simulink subsystem "RoboticArmGeneral7DOF_2"  (R2023a)
settings: Solver=VariableStepAuto  StartTime=0.0  StopTime=10.0  RelTol=1e-3
model mask{armAttach_Data=0, joint1_Data=0, joint2_Data=0, joint3_Data=0, joint4_Data=0, joint5_Data=0, joint6_Data=0, joint7_Data=0, ee_State_Data=0}
undefined symbols (not defined in the file or in its folder): arm, X, Y, Z
libraries: sm_lib x62, nesl_utility x35
(part 2 of 2)

== system RoboticArmGeneral7DOF_2/ElbowAssem_1/MainLink2_1_RIGID ==
  ReferenceFrame : sm_lib/Frames and Transforms/Reference Frame
  Solid : sm_lib/Body Elements/File Solid  ExtGeomFileName=MainLink2_Default_sldprt.STEP  UnitType=FromFile  ExtGeomFileUnits=m  StepReaderType=HEX  ExportConvexHullGeometry=off  InertiaType=Custom  Mass=arm(2).smiData.Solid(3).mass  MassUnits=kg  CenterOfMass=arm(2).smiData.Solid(3).CoM  CenterOfMassUnits=m  MomentsOfInertia=arm(2).smiData.Solid(3).MoI  MomentsOfInertiaUnits=kg*m^2  ProductsOfInertia=arm(2).smiData.Solid(3).PoI  ProductsOfInertiaUnits=kg*m^2  BasedOnType=DensityFromFile  Density=1000  DensityUnits=kg/m^3  DoExposeReferenceFrame=on  SerializedFrames=<Frames/>  GraphicType=FromGeometry  MarkerShape=Sphere  MarkerSize=10  GraphicVisPropType=SimpleVisualProperties  GraphicDiffuseColor=arm(2).smiData.Solid(3).color  GraphicSpecularColor=[0.5 0.5 0.5 1.0]  GraphicAmbientColor=[0.15 0.15 0.15 1.0]  GraphicEmissiveColor=[0.0 0.0 0.0 1.0]  GraphicShininess=75  GraphicOpacity=arm(2).smiData.Solid(3).opacity
  Transform : sm_lib/Frames and Transforms/Rigid Transform  TranslationMethod=Cartesian  TranslationStandardOffset=0  TranslationStandardOffsetUnits=m  TranslationStandardAxis=+Z  TranslationCartesianOffset=arm(2).smiData.RigidTransform(5).translation  TranslationCartesianOffsetUnits=m  TranslationROffset=0  TranslationROffsetUnits=m  TranslationZOffset=0  TranslationZOffsetUnits=m  TranslationThetaOffset=0  TranslationThetaOffsetUnits=deg  RotationMethod=ArbitraryAxis  RotationAngleUnits=rad  RotationStandardAxis=+Z  RotationAngle=arm(2).smiData.RigidTransform(5).angle  RotationArbitraryAxis=arm(2).smiData.RigidTransform(5).axis  FollAlignAxisA=+X  BaseAlignAxisA=+Y  FollAlignAxisB=+Y  BaseAlignAxisB=+Z  RotationSequenceAxes=FollowerAxes  RotationSequence=XYX  RotationSequenceAngles=[0 0 0]  RotationSequenceAnglesUnits=deg  RotationMatrix=[1 0 0; 0 1 0; 0 0 1]  Quaternion=[1 0 0 0]
  Transform1 : sm_lib/Frames and Transforms/Rigid Transform  TranslationMethod=Cartesian  TranslationStandardOffset=0  TranslationStandardOffsetUnits=m  TranslationStandardAxis=+Z  TranslationCartesianOffset=arm(2).smiData.RigidTransform(19).translation  TranslationCartesianOffsetUnits=m  TranslationROffset=0  TranslationROffsetUnits=m  TranslationZOffset=0  TranslationZOffsetUnits=m  TranslationThetaOffset=0  TranslationThetaOffsetUnits=deg  RotationMethod=ArbitraryAxis  RotationAngleUnits=rad  RotationStandardAxis=+Z  RotationAngle=arm(2).smiData.RigidTransform(19).angle  RotationArbitraryAxis=arm(2).smiData.RigidTransform(19).axis  FollAlignAxisA=+X  BaseAlignAxisA=+Y  FollAlignAxisB=+Y  BaseAlignAxisB=+Z  RotationSequenceAxes=FollowerAxes  RotationSequence=XYX  RotationSequenceAngles=[0 0 0]  RotationSequenceAnglesUnits=deg  RotationMatrix=[1 0 0; 0 1 0; 0 0 1]  Quaternion=[1 0 0 0]
  MainLink_End : PMIOPort  Side=Right
  J5_2 : PMIOPort  Port=2  Side=Left
  connections:
  Transform1/RConn1 -- MainLink_End/RConn1
  Transform/RConn1 -- J5_2/RConn1
  Transform1/LConn1 -- Transform/LConn1 -- ReferenceFrame/RConn1 -- Solid/RConn1

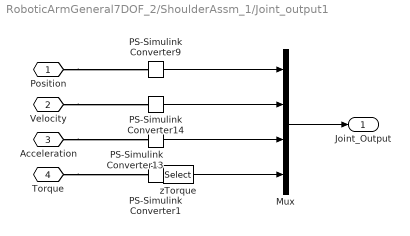
== system RoboticArmGeneral7DOF_2/ShoulderAssm_1/Joint_output1 ==
  Mux : Mux
  PS-Simulink Converter{1,9,13..14} (4 alike) : nesl_utility/PS-Simulink Converter  PhysicalDomain=network_engine_domain  SubClassName=ps_output  LeftPortType=input  RightPortType=output  PseudoPeriodic=off  Frequencies=[]  VectorFormat=1-D array  Unit=inherit  AffineConversion=off
  zTorque : Selector  InputPortWidth=3  IndexOptions=Index vector (dialog)  Indices=3  OutputSizes=1
  Position : PMIOPort  Side=Left
  Velocity : PMIOPort  Port=2  Side=Left
  Acceleration : PMIOPort  Port=3  Side=Left
  Torque : PMIOPort  Port=4  Side=Left
  Joint_Output : Outport
  wires:
  PS-Simulink Converter1/1 -> zTorque/1
  PS-Simulink Converter13/1 -> Mux/3
  PS-Simulink Converter9/1 -> Mux/1
  zTorque/1 -> Mux/4
  PS-Simulink Converter14/1 -> Mux/2
  Mux/1 -> Joint_Output/1
  connections:
  Position/RConn1 -- PS-Simulink Converter9/LConn1
  Acceleration/RConn1 -- PS-Simulink Converter13/LConn1
  Torque/RConn1 -- PS-Simulink Converter1/LConn1
  Velocity/RConn1 -- PS-Simulink Converter14/LConn1

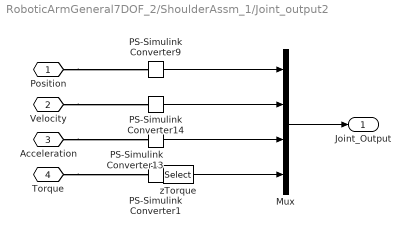
== system RoboticArmGeneral7DOF_2/ShoulderAssm_1/Joint_output2 ==
  Mux : Mux
  PS-Simulink Converter{1,9,13..14} (4 alike) : nesl_utility/PS-Simulink Converter  PhysicalDomain=network_engine_domain  SubClassName=ps_output  LeftPortType=input  RightPortType=output  PseudoPeriodic=off  Frequencies=[]  VectorFormat=1-D array  Unit=inherit  AffineConversion=off
  zTorque : Selector  InputPortWidth=3  IndexOptions=Index vector (dialog)  Indices=3  OutputSizes=1
  Position : PMIOPort  Side=Left
  Velocity : PMIOPort  Port=2  Side=Left
  Acceleration : PMIOPort  Port=3  Side=Left
  Torque : PMIOPort  Port=4  Side=Left
  Joint_Output : Outport
  wires:
  PS-Simulink Converter1/1 -> zTorque/1
  PS-Simulink Converter13/1 -> Mux/3
  PS-Simulink Converter9/1 -> Mux/1
  zTorque/1 -> Mux/4
  PS-Simulink Converter14/1 -> Mux/2
  Mux/1 -> Joint_Output/1
  connections:
  Position/RConn1 -- PS-Simulink Converter9/LConn1
  Acceleration/RConn1 -- PS-Simulink Converter13/LConn1
  Torque/RConn1 -- PS-Simulink Converter1/LConn1
  Velocity/RConn1 -- PS-Simulink Converter14/LConn1

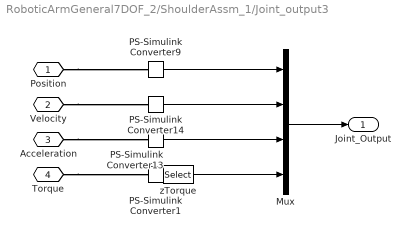
== system RoboticArmGeneral7DOF_2/ShoulderAssm_1/Joint_output3 ==
  Mux : Mux
  PS-Simulink Converter{1,9,13..14} (4 alike) : nesl_utility/PS-Simulink Converter  PhysicalDomain=network_engine_domain  SubClassName=ps_output  LeftPortType=input  RightPortType=output  PseudoPeriodic=off  Frequencies=[]  VectorFormat=1-D array  Unit=inherit  AffineConversion=off
  zTorque : Selector  InputPortWidth=3  IndexOptions=Index vector (dialog)  Indices=3  OutputSizes=1
  Position : PMIOPort  Side=Left
  Velocity : PMIOPort  Port=2  Side=Left
  Acceleration : PMIOPort  Port=3  Side=Left
  Torque : PMIOPort  Port=4  Side=Left
  Joint_Output : Outport
  wires:
  PS-Simulink Converter1/1 -> zTorque/1
  PS-Simulink Converter13/1 -> Mux/3
  PS-Simulink Converter9/1 -> Mux/1
  zTorque/1 -> Mux/4
  PS-Simulink Converter14/1 -> Mux/2
  Mux/1 -> Joint_Output/1
  connections:
  Position/RConn1 -- PS-Simulink Converter9/LConn1
  Acceleration/RConn1 -- PS-Simulink Converter13/LConn1
  Torque/RConn1 -- PS-Simulink Converter1/LConn1
  Velocity/RConn1 -- PS-Simulink Converter14/LConn1

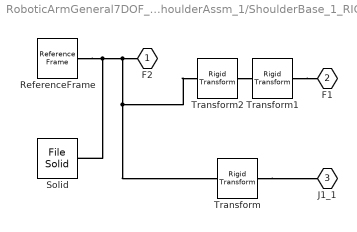
== system RoboticArmGeneral7DOF_2/ShoulderAssm_1/ShoulderBase_1_RIGID ==
  ReferenceFrame : sm_lib/Frames and Transforms/Reference Frame
  Solid : sm_lib/Body Elements/File Solid  ExtGeomFileName=ShoulderBase_Default_sldprt.STEP  UnitType=FromFile  ExtGeomFileUnits=m  StepReaderType=HEX  ExportConvexHullGeometry=off  InertiaType=Custom  Mass=arm(2).smiData.Solid(9).mass  MassUnits=kg  CenterOfMass=arm(2).smiData.Solid(9).CoM  CenterOfMassUnits=m  MomentsOfInertia=arm(2).smiData.Solid(9).MoI  MomentsOfInertiaUnits=kg*m^2  ProductsOfInertia=arm(2).smiData.Solid(9).PoI  ProductsOfInertiaUnits=kg*m^2  BasedOnType=DensityFromFile  Density=1000  DensityUnits=kg/m^3  DoExposeReferenceFrame=on  SerializedFrames=<Frames/>  GraphicType=FromGeometry  MarkerShape=Sphere  MarkerSize=10  GraphicVisPropType=SimpleVisualProperties  GraphicDiffuseColor=arm(2).smiData.Solid(9).color  GraphicSpecularColor=[0.5 0.5 0.5 1.0]  GraphicAmbientColor=[0.15 0.15 0.15 1.0]  GraphicEmissiveColor=[0.0 0.0 0.0 1.0]  GraphicShininess=75  GraphicOpacity=arm(2).smiData.Solid(9).opacity
  Transform : sm_lib/Frames and Transforms/Rigid Transform  TranslationMethod=Cartesian  TranslationStandardOffset=0  TranslationStandardOffsetUnits=m  TranslationStandardAxis=+Z  TranslationCartesianOffset=arm(2).smiData.RigidTransform(9).translation  TranslationCartesianOffsetUnits=m  TranslationROffset=0  TranslationROffsetUnits=m  TranslationZOffset=0  TranslationZOffsetUnits=m  TranslationThetaOffset=0  TranslationThetaOffsetUnits=deg  RotationMethod=ArbitraryAxis  RotationAngleUnits=rad  RotationStandardAxis=+Z  RotationAngle=arm(2).smiData.RigidTransform(9).angle  RotationArbitraryAxis=arm(2).smiData.RigidTransform(9).axis  FollAlignAxisA=+X  BaseAlignAxisA=+Y  FollAlignAxisB=+Y  BaseAlignAxisB=+Z  RotationSequenceAxes=FollowerAxes  RotationSequence=XYX  RotationSequenceAngles=[0 0 0]  RotationSequenceAnglesUnits=deg  RotationMatrix=[1 0 0; 0 1 0; 0 0 1]  Quaternion=[1 0 0 0]
  Transform1 : sm_lib/Frames and Transforms/Rigid Transform  TranslationMethod=Cartesian  TranslationStandardOffset=0  TranslationStandardOffsetUnits=m  TranslationStandardAxis=+Z  TranslationCartesianOffset=arm(2).smiData.RigidTransform(15).translation  TranslationCartesianOffsetUnits=m  TranslationROffset=0  TranslationROffsetUnits=m  TranslationZOffset=0  TranslationZOffsetUnits=m  TranslationThetaOffset=0  TranslationThetaOffsetUnits=deg  RotationMethod=ArbitraryAxis  RotationAngleUnits=rad  RotationStandardAxis=+Z  RotationAngle=arm(2).smiData.RigidTransform(15).angle  RotationArbitraryAxis=arm(2).smiData.RigidTransform(15).axis  FollAlignAxisA=+X  BaseAlignAxisA=+Y  FollAlignAxisB=+Y  BaseAlignAxisB=+Z  RotationSequenceAxes=FollowerAxes  RotationSequence=XYX  RotationSequenceAngles=[0 0 0]  RotationSequenceAnglesUnits=deg  RotationMatrix=[1 0 0; 0 1 0; 0 0 1]  Quaternion=[1 0 0 0]
  Transform2 : sm_lib/Frames and Transforms/Rigid Transform  TranslationMethod=Cartesian  TranslationStandardOffset=0  TranslationStandardOffsetUnits=m  TranslationStandardAxis=+Z  TranslationCartesianOffset=arm(2).smiData.RigidTransform(25).translation  TranslationCartesianOffsetUnits=m  TranslationROffset=0  TranslationROffsetUnits=m  TranslationZOffset=0  TranslationZOffsetUnits=m  TranslationThetaOffset=0  TranslationThetaOffsetUnits=deg  RotationMethod=ArbitraryAxis  RotationAngleUnits=rad  RotationStandardAxis=+Z  RotationAngle=arm(2).smiData.RigidTransform(25).angle  RotationArbitraryAxis=arm(2).smiData.RigidTransform(25).axis  FollAlignAxisA=+X  BaseAlignAxisA=+Y  FollAlignAxisB=+Y  BaseAlignAxisB=+Z  RotationSequenceAxes=FollowerAxes  RotationSequence=XYX  RotationSequenceAngles=[0 0 0]  RotationSequenceAnglesUnits=deg  RotationMatrix=[1 0 0; 0 1 0; 0 0 1]  Quaternion=[1 0 0 0]
  F2 : PMIOPort  Side=Left
  F1 : PMIOPort  Port=2  Side=Left
  J1_1 : PMIOPort  Port=3  Side=Right
  connections:
  Transform2/LConn1 -- Transform/LConn1 -- F2/RConn1 -- ReferenceFrame/RConn1 -- Solid/RConn1
  Transform1/RConn1 -- F1/RConn1
  Transform/RConn1 -- J1_1/RConn1
  Transform2/RConn1 -- Transform1/LConn1

== system RoboticArmGeneral7DOF_2/ShoulderAssm_1/ShoulderJoint_1_1_RIGID ==
  ReferenceFrame : sm_lib/Frames and Transforms/Reference Frame
  Solid : sm_lib/Body Elements/File Solid  ExtGeomFileName=ShoulderJoint_1_Default_sldprt.STEP  UnitType=FromFile  ExtGeomFileUnits=m  StepReaderType=HEX  ExportConvexHullGeometry=off  InertiaType=Custom  Mass=arm(2).smiData.Solid(7).mass  MassUnits=kg  CenterOfMass=arm(2).smiData.Solid(7).CoM  CenterOfMassUnits=m  MomentsOfInertia=arm(2).smiData.Solid(7).MoI  MomentsOfInertiaUnits=kg*m^2  ProductsOfInertia=arm(2).smiData.Solid(7).PoI  ProductsOfInertiaUnits=kg*m^2  BasedOnType=DensityFromFile  Density=1000  DensityUnits=kg/m^3  DoExposeReferenceFrame=on  SerializedFrames=<Frames/>  GraphicType=FromGeometry  MarkerShape=Sphere  MarkerSize=10  GraphicVisPropType=SimpleVisualProperties  GraphicDiffuseColor=arm(2).smiData.Solid(7).color  GraphicSpecularColor=[0.5 0.5 0.5 1.0]  GraphicAmbientColor=[0.15 0.15 0.15 1.0]  GraphicEmissiveColor=[0.0 0.0 0.0 1.0]  GraphicShininess=75  GraphicOpacity=arm(2).smiData.Solid(7).opacity
  Transform : sm_lib/Frames and Transforms/Rigid Transform  TranslationMethod=Cartesian  TranslationStandardOffset=0  TranslationStandardOffsetUnits=m  TranslationStandardAxis=+Z  TranslationCartesianOffset=arm(2).smiData.RigidTransform(10).translation  TranslationCartesianOffsetUnits=m  TranslationROffset=0  TranslationROffsetUnits=m  TranslationZOffset=0  TranslationZOffsetUnits=m  TranslationThetaOffset=0  TranslationThetaOffsetUnits=deg  RotationMethod=ArbitraryAxis  RotationAngleUnits=rad  RotationStandardAxis=+Z  RotationAngle=arm(2).smiData.RigidTransform(10).angle  RotationArbitraryAxis=arm(2).smiData.RigidTransform(10).axis  FollAlignAxisA=+X  BaseAlignAxisA=+Y  FollAlignAxisB=+Y  BaseAlignAxisB=+Z  RotationSequenceAxes=FollowerAxes  RotationSequence=XYX  RotationSequenceAngles=[0 0 0]  RotationSequenceAnglesUnits=deg  RotationMatrix=[1 0 0; 0 1 0; 0 0 1]  Quaternion=[1 0 0 0]
  Transform1 : sm_lib/Frames and Transforms/Rigid Transform  TranslationMethod=Cartesian  TranslationStandardOffset=0  TranslationStandardOffsetUnits=m  TranslationStandardAxis=+Z  TranslationCartesianOffset=arm(2).smiData.RigidTransform(11).translation  TranslationCartesianOffsetUnits=m  TranslationROffset=0  TranslationROffsetUnits=m  TranslationZOffset=0  TranslationZOffsetUnits=m  TranslationThetaOffset=0  TranslationThetaOffsetUnits=deg  RotationMethod=ArbitraryAxis  RotationAngleUnits=rad  RotationStandardAxis=+Z  RotationAngle=arm(2).smiData.RigidTransform(11).angle  RotationArbitraryAxis=arm(2).smiData.RigidTransform(11).axis  FollAlignAxisA=+X  BaseAlignAxisA=+Y  FollAlignAxisB=+Y  BaseAlignAxisB=+Z  RotationSequenceAxes=FollowerAxes  RotationSequence=XYX  RotationSequenceAngles=[0 0 0]  RotationSequenceAnglesUnits=deg  RotationMatrix=[1 0 0; 0 1 0; 0 0 1]  Quaternion=[1 0 0 0]
  Shoulder1 : PMIOPort  Side=Right
  J1_2 : PMIOPort  Port=2  Side=Left
  AfterT : PMIOPort  Port=3  Side=Left
  connections:
  Shoulder1/RConn1 -- Transform1/RConn1
  Transform/RConn1 -- J1_2/RConn1
  AfterT/RConn1 -- Transform1/LConn1 -- ReferenceFrame/RConn1 -- Solid/RConn1 -- Transform/LConn1

== system RoboticArmGeneral7DOF_2/ShoulderAssm_1/ShoulderJoint_2_1_RIGID ==
  ReferenceFrame : sm_lib/Frames and Transforms/Reference Frame
  Solid : sm_lib/Body Elements/File Solid  ExtGeomFileName=ShoulderJoint_2_Default_sldprt.STEP  UnitType=FromFile  ExtGeomFileUnits=m  StepReaderType=HEX  ExportConvexHullGeometry=off  InertiaType=Custom  Mass=arm(2).smiData.Solid(8).mass  MassUnits=kg  CenterOfMass=arm(2).smiData.Solid(8).CoM  CenterOfMassUnits=m  MomentsOfInertia=arm(2).smiData.Solid(8).MoI  MomentsOfInertiaUnits=kg*m^2  ProductsOfInertia=arm(2).smiData.Solid(8).PoI  ProductsOfInertiaUnits=kg*m^2  BasedOnType=DensityFromFile  Density=1000  DensityUnits=kg/m^3  DoExposeReferenceFrame=on  SerializedFrames=<Frames/>  GraphicType=FromGeometry  MarkerShape=Sphere  MarkerSize=10  GraphicVisPropType=SimpleVisualProperties  GraphicDiffuseColor=arm(2).smiData.Solid(8).color  GraphicSpecularColor=[0.5 0.5 0.5 1.0]  GraphicAmbientColor=[0.15 0.15 0.15 1.0]  GraphicEmissiveColor=[0.0 0.0 0.0 1.0]  GraphicShininess=75  GraphicOpacity=arm(2).smiData.Solid(8).opacity
  Transform : sm_lib/Frames and Transforms/Rigid Transform  TranslationMethod=Cartesian  TranslationStandardOffset=0  TranslationStandardOffsetUnits=m  TranslationStandardAxis=+Z  TranslationCartesianOffset=arm(2).smiData.RigidTransform(12).translation  TranslationCartesianOffsetUnits=m  TranslationROffset=0  TranslationROffsetUnits=m  TranslationZOffset=0  TranslationZOffsetUnits=m  TranslationThetaOffset=0  TranslationThetaOffsetUnits=deg  RotationMethod=ArbitraryAxis  RotationAngleUnits=rad  RotationStandardAxis=+Z  RotationAngle=arm(2).smiData.RigidTransform(12).angle  RotationArbitraryAxis=arm(2).smiData.RigidTransform(12).axis  FollAlignAxisA=+X  BaseAlignAxisA=+Y  FollAlignAxisB=+Y  BaseAlignAxisB=+Z  RotationSequenceAxes=FollowerAxes  RotationSequence=XYX  RotationSequenceAngles=[0 0 0]  RotationSequenceAnglesUnits=deg  RotationMatrix=[1 0 0; 0 1 0; 0 0 1]  Quaternion=[1 0 0 0]
  Transform1 : sm_lib/Frames and Transforms/Rigid Transform  TranslationMethod=Cartesian  TranslationStandardOffset=0  TranslationStandardOffsetUnits=m  TranslationStandardAxis=+Z  TranslationCartesianOffset=arm(2).smiData.RigidTransform(13).translation  TranslationCartesianOffsetUnits=m  TranslationROffset=0  TranslationROffsetUnits=m  TranslationZOffset=0  TranslationZOffsetUnits=m  TranslationThetaOffset=0  TranslationThetaOffsetUnits=deg  RotationMethod=ArbitraryAxis  RotationAngleUnits=rad  RotationStandardAxis=+Z  RotationAngle=arm(2).smiData.RigidTransform(13).angle  RotationArbitraryAxis=arm(2).smiData.RigidTransform(13).axis  FollAlignAxisA=+X  BaseAlignAxisA=+Y  FollAlignAxisB=+Y  BaseAlignAxisB=+Z  RotationSequenceAxes=FollowerAxes  RotationSequence=XYX  RotationSequenceAngles=[0 0 0]  RotationSequenceAnglesUnits=deg  RotationMatrix=[1 0 0; 0 1 0; 0 0 1]  Quaternion=[1 0 0 0]
  J2_1 : PMIOPort  Side=Right
  Shoulder1 : PMIOPort  Port=2  Side=Left
  connections:
  Transform1/RConn1 -- J2_1/RConn1
  Transform/RConn1 -- Shoulder1/RConn1
  Solid/RConn1 -- Transform1/LConn1 -- Transform/LConn1 -- ReferenceFrame/RConn1

== system RoboticArmGeneral7DOF_2/ShoulderAssm_1/ShoulderJoint_3_4_RIGID ==
  ReferenceFrame : sm_lib/Frames and Transforms/Reference Frame
  Solid : sm_lib/Body Elements/File Solid  ExtGeomFileName=ShoulderJoint_3_Default_sldprt.STEP  UnitType=FromFile  ExtGeomFileUnits=m  StepReaderType=HEX  ExportConvexHullGeometry=off  InertiaType=Custom  Mass=arm(2).smiData.Solid(10).mass  MassUnits=kg  CenterOfMass=arm(2).smiData.Solid(10).CoM  CenterOfMassUnits=m  MomentsOfInertia=arm(2).smiData.Solid(10).MoI  MomentsOfInertiaUnits=kg*m^2  ProductsOfInertia=arm(2).smiData.Solid(10).PoI  ProductsOfInertiaUnits=kg*m^2  BasedOnType=DensityFromFile  Density=1000  DensityUnits=kg/m^3  DoExposeReferenceFrame=on  SerializedFrames=<Frames/>  GraphicType=FromGeometry  MarkerShape=Sphere  MarkerSize=10  GraphicVisPropType=SimpleVisualProperties  GraphicDiffuseColor=arm(2).smiData.Solid(10).color  GraphicSpecularColor=[0.5 0.5 0.5 1.0]  GraphicAmbientColor=[0.15 0.15 0.15 1.0]  GraphicEmissiveColor=[0.0 0.0 0.0 1.0]  GraphicShininess=75  GraphicOpacity=arm(2).smiData.Solid(10).opacity
  Transform : sm_lib/Frames and Transforms/Rigid Transform  TranslationMethod=Cartesian  TranslationStandardOffset=0  TranslationStandardOffsetUnits=m  TranslationStandardAxis=+Z  TranslationCartesianOffset=arm(2).smiData.RigidTransform(14).translation  TranslationCartesianOffsetUnits=m  TranslationROffset=0  TranslationROffsetUnits=m  TranslationZOffset=0  TranslationZOffsetUnits=m  TranslationThetaOffset=0  TranslationThetaOffsetUnits=deg  RotationMethod=ArbitraryAxis  RotationAngleUnits=rad  RotationStandardAxis=+Z  RotationAngle=arm(2).smiData.RigidTransform(14).angle  RotationArbitraryAxis=arm(2).smiData.RigidTransform(14).axis  FollAlignAxisA=+X  BaseAlignAxisA=+Y  FollAlignAxisB=+Y  BaseAlignAxisB=+Z  RotationSequenceAxes=FollowerAxes  RotationSequence=XYX  RotationSequenceAngles=[0 0 0]  RotationSequenceAnglesUnits=deg  RotationMatrix=[1 0 0; 0 1 0; 0 0 1]  Quaternion=[1 0 0 0]
  Transform1 : sm_lib/Frames and Transforms/Rigid Transform  TranslationMethod=Cartesian  TranslationStandardOffset=0  TranslationStandardOffsetUnits=m  TranslationStandardAxis=+Z  TranslationCartesianOffset=arm(2).smiData.RigidTransform(21).translation  TranslationCartesianOffsetUnits=m  TranslationROffset=0  TranslationROffsetUnits=m  TranslationZOffset=0  TranslationZOffsetUnits=m  TranslationThetaOffset=0  TranslationThetaOffsetUnits=deg  RotationMethod=ArbitraryAxis  RotationAngleUnits=rad  RotationStandardAxis=+Z  RotationAngle=arm(2).smiData.RigidTransform(21).angle  RotationArbitraryAxis=arm(2).smiData.RigidTransform(21).axis  FollAlignAxisA=+X  BaseAlignAxisA=+Y  FollAlignAxisB=+Y  BaseAlignAxisB=+Z  RotationSequenceAxes=FollowerAxes  RotationSequence=XYX  RotationSequenceAngles=[0 0 0]  RotationSequenceAnglesUnits=deg  RotationMatrix=[1 0 0; 0 1 0; 0 0 1]  Quaternion=[1 0 0 0]
  J3_1 : PMIOPort  Side=Right
  J2_2 : PMIOPort  Port=2  Side=Left
  connections:
  Transform1/RConn1 -- J3_1/RConn1
  Transform/RConn1 -- J2_2/RConn1
  Transform1/LConn1 -- Transform/LConn1 -- ReferenceFrame/RConn1 -- Solid/RConn1

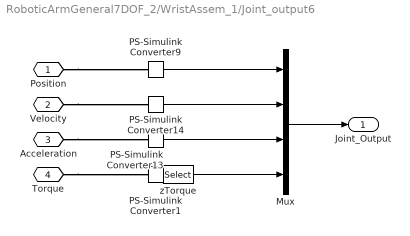
== system RoboticArmGeneral7DOF_2/WristAssem_1/Joint_output6 ==
  Mux : Mux
  PS-Simulink Converter{1,9,13..14} (4 alike) : nesl_utility/PS-Simulink Converter  PhysicalDomain=network_engine_domain  SubClassName=ps_output  LeftPortType=input  RightPortType=output  PseudoPeriodic=off  Frequencies=[]  VectorFormat=1-D array  Unit=inherit  AffineConversion=off
  zTorque : Selector  InputPortWidth=3  IndexOptions=Index vector (dialog)  Indices=3  OutputSizes=1
  Position : PMIOPort  Side=Left
  Velocity : PMIOPort  Port=2  Side=Left
  Acceleration : PMIOPort  Port=3  Side=Left
  Torque : PMIOPort  Port=4  Side=Left
  Joint_Output : Outport
  wires:
  PS-Simulink Converter1/1 -> zTorque/1
  PS-Simulink Converter13/1 -> Mux/3
  PS-Simulink Converter9/1 -> Mux/1
  zTorque/1 -> Mux/4
  PS-Simulink Converter14/1 -> Mux/2
  Mux/1 -> Joint_Output/1
  connections:
  Position/RConn1 -- PS-Simulink Converter9/LConn1
  Acceleration/RConn1 -- PS-Simulink Converter13/LConn1
  Torque/RConn1 -- PS-Simulink Converter1/LConn1
  Velocity/RConn1 -- PS-Simulink Converter14/LConn1

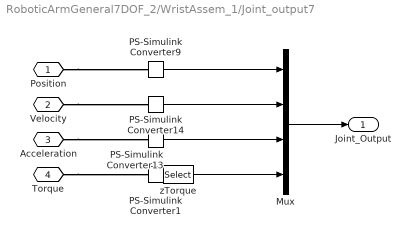
== system RoboticArmGeneral7DOF_2/WristAssem_1/Joint_output7 ==
  Mux : Mux
  PS-Simulink Converter{1,9,13..14} (4 alike) : nesl_utility/PS-Simulink Converter  PhysicalDomain=network_engine_domain  SubClassName=ps_output  LeftPortType=input  RightPortType=output  PseudoPeriodic=off  Frequencies=[]  VectorFormat=1-D array  Unit=inherit  AffineConversion=off
  zTorque : Selector  InputPortWidth=3  IndexOptions=Index vector (dialog)  Indices=3  OutputSizes=1
  Position : PMIOPort  Side=Left
  Velocity : PMIOPort  Port=2  Side=Left
  Acceleration : PMIOPort  Port=3  Side=Left
  Torque : PMIOPort  Port=4  Side=Left
  Joint_Output : Outport
  wires:
  PS-Simulink Converter1/1 -> zTorque/1
  PS-Simulink Converter13/1 -> Mux/3
  PS-Simulink Converter9/1 -> Mux/1
  zTorque/1 -> Mux/4
  PS-Simulink Converter14/1 -> Mux/2
  Mux/1 -> Joint_Output/1
  connections:
  Position/RConn1 -- PS-Simulink Converter9/LConn1
  Acceleration/RConn1 -- PS-Simulink Converter13/LConn1
  Torque/RConn1 -- PS-Simulink Converter1/LConn1
  Velocity/RConn1 -- PS-Simulink Converter14/LConn1

== system RoboticArmGeneral7DOF_2/WristAssem_1/WristJoint_1_1_RIGID ==
  ReferenceFrame : sm_lib/Frames and Transforms/Reference Frame
  Solid : sm_lib/Body Elements/File Solid  ExtGeomFileName=WristJoint_1_Default_sldprt.STEP  UnitType=FromFile  ExtGeomFileUnits=m  StepReaderType=HEX  ExportConvexHullGeometry=off  InertiaType=Custom  Mass=arm(2).smiData.Solid(5).mass  MassUnits=kg  CenterOfMass=arm(2).smiData.Solid(5).CoM  CenterOfMassUnits=m  MomentsOfInertia=arm(2).smiData.Solid(5).MoI  MomentsOfInertiaUnits=kg*m^2  ProductsOfInertia=arm(2).smiData.Solid(5).PoI  ProductsOfInertiaUnits=kg*m^2  BasedOnType=DensityFromFile  Density=1000  DensityUnits=kg/m^3  DoExposeReferenceFrame=on  SerializedFrames=<Frames/>  GraphicType=FromGeometry  MarkerShape=Sphere  MarkerSize=10  GraphicVisPropType=SimpleVisualProperties  GraphicDiffuseColor=arm(2).smiData.Solid(5).color  GraphicSpecularColor=[0.5 0.5 0.5 1.0]  GraphicAmbientColor=[0.15 0.15 0.15 1.0]  GraphicEmissiveColor=[0.0 0.0 0.0 1.0]  GraphicShininess=75  GraphicOpacity=arm(2).smiData.Solid(5).opacity
  Transform : sm_lib/Frames and Transforms/Rigid Transform  TranslationMethod=Cartesian  TranslationStandardOffset=0  TranslationStandardOffsetUnits=m  TranslationStandardAxis=+Z  TranslationCartesianOffset=arm(2).smiData.RigidTransform(7).translation  TranslationCartesianOffsetUnits=m  TranslationROffset=0  TranslationROffsetUnits=m  TranslationZOffset=0  TranslationZOffsetUnits=m  TranslationThetaOffset=0  TranslationThetaOffsetUnits=deg  RotationMethod=ArbitraryAxis  RotationAngleUnits=rad  RotationStandardAxis=+Z  RotationAngle=arm(2).smiData.RigidTransform(7).angle  RotationArbitraryAxis=arm(2).smiData.RigidTransform(7).axis  FollAlignAxisA=+X  BaseAlignAxisA=+Y  FollAlignAxisB=+Y  BaseAlignAxisB=+Z  RotationSequenceAxes=FollowerAxes  RotationSequence=XYX  RotationSequenceAngles=[0 0 0]  RotationSequenceAnglesUnits=deg  RotationMatrix=[1 0 0; 0 1 0; 0 0 1]  Quaternion=[1 0 0 0]
  Transform1 : sm_lib/Frames and Transforms/Rigid Transform  TranslationMethod=Cartesian  TranslationStandardOffset=0  TranslationStandardOffsetUnits=m  TranslationStandardAxis=+Z  TranslationCartesianOffset=arm(2).smiData.RigidTransform(20).translation  TranslationCartesianOffsetUnits=m  TranslationROffset=0  TranslationROffsetUnits=m  TranslationZOffset=0  TranslationZOffsetUnits=m  TranslationThetaOffset=0  TranslationThetaOffsetUnits=deg  RotationMethod=ArbitraryAxis  RotationAngleUnits=rad  RotationStandardAxis=+Z  RotationAngle=arm(2).smiData.RigidTransform(20).angle  RotationArbitraryAxis=arm(2).smiData.RigidTransform(20).axis  FollAlignAxisA=+X  BaseAlignAxisA=+Y  FollAlignAxisB=+Y  BaseAlignAxisB=+Z  RotationSequenceAxes=FollowerAxes  RotationSequence=XYX  RotationSequenceAngles=[0 0 0]  RotationSequenceAnglesUnits=deg  RotationMatrix=[1 0 0; 0 1 0; 0 0 1]  Quaternion=[1 0 0 0]
  J6_1 : PMIOPort  Side=Right
  F2 : PMIOPort  Port=2  Side=Left
  F1 : PMIOPort  Port=3  Side=Left
  connections:
  Transform1/RConn1 -- F1/RConn1
  Transform/RConn1 -- J6_1/RConn1
  F2/RConn1 -- Transform1/LConn1 -- Transform/LConn1 -- ReferenceFrame/RConn1 -- Solid/RConn1

== system RoboticArmGeneral7DOF_2/WristAssem_1/WristJoint_2_1_RIGID ==
  ReferenceFrame : sm_lib/Frames and Transforms/Reference Frame
  Solid : sm_lib/Body Elements/File Solid  ExtGeomFileName=WristJoint_2_Default_sldprt.STEP  UnitType=FromFile  ExtGeomFileUnits=m  StepReaderType=HEX  ExportConvexHullGeometry=off  InertiaType=Custom  Mass=arm(2).smiData.Solid(6).mass  MassUnits=kg  CenterOfMass=arm(2).smiData.Solid(6).CoM  CenterOfMassUnits=m  MomentsOfInertia=arm(2).smiData.Solid(6).MoI  MomentsOfInertiaUnits=kg*m^2  ProductsOfInertia=arm(2).smiData.Solid(6).PoI  ProductsOfInertiaUnits=kg*m^2  BasedOnType=DensityFromFile  Density=1000  DensityUnits=kg/m^3  DoExposeReferenceFrame=on  SerializedFrames=<Frames/>  GraphicType=FromGeometry  MarkerShape=Sphere  MarkerSize=10  GraphicVisPropType=SimpleVisualProperties  GraphicDiffuseColor=arm(2).smiData.Solid(6).color  GraphicSpecularColor=[0.5 0.5 0.5 1.0]  GraphicAmbientColor=[0.15 0.15 0.15 1.0]  GraphicEmissiveColor=[0.0 0.0 0.0 1.0]  GraphicShininess=75  GraphicOpacity=arm(2).smiData.Solid(6).opacity
  Transform : sm_lib/Frames and Transforms/Rigid Transform  TranslationMethod=Cartesian  TranslationStandardOffset=0  TranslationStandardOffsetUnits=m  TranslationStandardAxis=+Z  TranslationCartesianOffset=arm(2).smiData.RigidTransform(8).translation  TranslationCartesianOffsetUnits=m  TranslationROffset=0  TranslationROffsetUnits=m  TranslationZOffset=0  TranslationZOffsetUnits=m  TranslationThetaOffset=0  TranslationThetaOffsetUnits=deg  RotationMethod=ArbitraryAxis  RotationAngleUnits=rad  RotationStandardAxis=+Z  RotationAngle=arm(2).smiData.RigidTransform(8).angle  RotationArbitraryAxis=arm(2).smiData.RigidTransform(8).axis  FollAlignAxisA=+X  BaseAlignAxisA=+Y  FollAlignAxisB=+Y  BaseAlignAxisB=+Z  RotationSequenceAxes=FollowerAxes  RotationSequence=XYX  RotationSequenceAngles=[0 0 0]  RotationSequenceAnglesUnits=deg  RotationMatrix=[1 0 0; 0 1 0; 0 0 1]  Quaternion=[1 0 0 0]
  Transform1 : sm_lib/Frames and Transforms/Rigid Transform  TranslationMethod=Cartesian  TranslationStandardOffset=0  TranslationStandardOffsetUnits=m  TranslationStandardAxis=+Z  TranslationCartesianOffset=arm(2).smiData.RigidTransform(17).translation  TranslationCartesianOffsetUnits=m  TranslationROffset=0  TranslationROffsetUnits=m  TranslationZOffset=0  TranslationZOffsetUnits=m  TranslationThetaOffset=0  TranslationThetaOffsetUnits=deg  RotationMethod=ArbitraryAxis  RotationAngleUnits=rad  RotationStandardAxis=+Z  RotationAngle=arm(2).smiData.RigidTransform(17).angle  RotationArbitraryAxis=arm(2).smiData.RigidTransform(17).axis  FollAlignAxisA=+X  BaseAlignAxisA=+Y  FollAlignAxisB=+Y  BaseAlignAxisB=+Z  RotationSequenceAxes=FollowerAxes  RotationSequence=XYX  RotationSequenceAngles=[0 0 0]  RotationSequenceAnglesUnits=deg  RotationMatrix=[1 0 0; 0 1 0; 0 0 1]  Quaternion=[1 0 0 0]
  J7_1 : PMIOPort  Side=Right
  J6_2 : PMIOPort  Port=2  Side=Left
  connections:
  Transform1/RConn1 -- J7_1/RConn1
  Transform/RConn1 -- J6_2/RConn1
  Transform1/LConn1 -- Transform/LConn1 -- ReferenceFrame/RConn1 -- Solid/RConn1
